simulink model "gm_untitled"  (R2020b)
settings: Solver=VariableStepAuto  StartTime=0.0  StopTime=0.001  RelTol=1e-3
libraries: simulink x1
settings Model: Creator=pablo  LastModifiedBy=pablo
settings OptimizationCC: BlockReduction=off  ConditionallyExecuteInputs=off
settings DebuggingCC: InheritedTsInSrcMsg=none

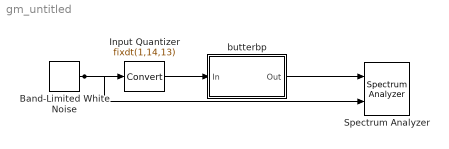
== system gm_untitled ==
  Band-Limited White Noise : simulink/Sources/Band-Limited White Noise  Cov=[0.1]  Ts=0.1  seed=[23341]
  Input Quantizer : DataTypeConversion  OutDataTypeStr=fixdt(1,14,13)  RndMeth=Round  SaturateOnIntegerOverflow=on
  Spectrum Analyzer : SpectrumAnalyzer  NumInputPorts=2
  butterbp : Subsystem
  wires:
  Band-Limited White Noise/1 -> Input Quantizer/1, Spectrum Analyzer/2
  butterbp/1(Out) -> Spectrum Analyzer/1
  Input Quantizer/1 -> butterbp/1(In)

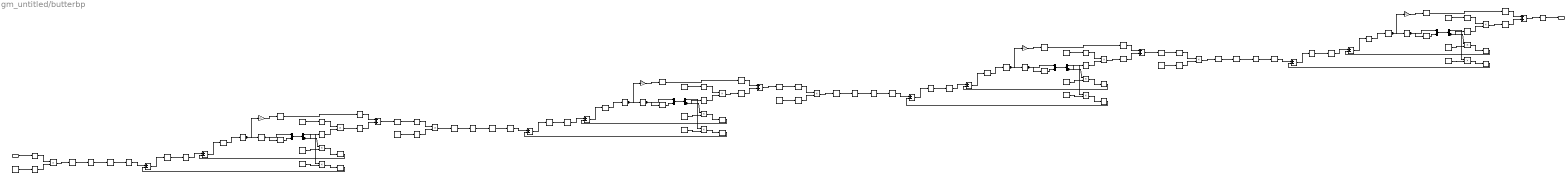
== system gm_untitled/butterbp ==
  In : Inport  OutDataTypeStr=fixdt(1, 14, 13)  PortDimensions=1  SampleTime=0.1
  HwModeRegister{,1..15} (16 alike) : Delay  DelayLength=double(1)  InitialCondition=0  SampleTime=0.1
  PipelineRegister{,1..7} (8 alike) : Delay  DelayLength=double(1)  InitialCondition=0  SampleTime=0.1
  Sub{,1..7} (8 alike) : Sum  Inputs=+-  OutDataTypeStr=fixdt(1, 41, 29)  RndMeth=Convergent  SampleTime=0.1
  adder{,1..3} (4 alike) : Sum  OutDataTypeStr=fixdt(1, 40, 29)  RndMeth=Convergent  SampleTime=0.1
  const : Constant  Value=0.009670734405517578125  OutDataTypeStr=fixdt(1, 16, 21)  SampleTime=0.1
  const1 : Constant  Value=-1.60137939453125  OutDataTypeStr=fixdt(1, 16, 14)  SampleTime=0.1
  const10 : Constant  Value=-1.60809326171875  OutDataTypeStr=fixdt(1, 16, 14)  SampleTime=0.1
  const11 : Constant  Value=0.9822998046875  OutDataTypeStr=fixdt(1, 16, 14)  SampleTime=0.1
  const2 : Constant  Value=0.99249267578125  OutDataTypeStr=fixdt(1, 16, 14)  SampleTime=0.1
  const3 : Constant  Value=0.009670734405517578125  OutDataTypeStr=fixdt(1, 16, 21)  SampleTime=0.1
  const4 : Constant  Value=-1.62249755859375  OutDataTypeStr=fixdt(1, 16, 14)  SampleTime=0.1
  const5 : Constant  Value=0.99267578125  OutDataTypeStr=fixdt(1, 16, 14)  SampleTime=0.1
  const6 : Constant  Value=0.00962066650390625  OutDataTypeStr=fixdt(1, 16, 21)  SampleTime=0.1
  const7 : Constant  Value=-1.5992431640625  OutDataTypeStr=fixdt(1, 16, 14)  SampleTime=0.1
  const8 : Constant  Value=0.98211669921875  OutDataTypeStr=fixdt(1, 16, 14)  SampleTime=0.1
  const9 : Constant  Value=0.00962066650390625  OutDataTypeStr=fixdt(1, 16, 21)  SampleTime=0.1
  delayMatch{,1..3} (4 alike) : Delay  DelayLength=double(2)  InitialCondition=0  SampleTime=0.1
  delay_process_section1_tap0 : Delay  DelayLength=double(1)  SampleTime=0.1
  delay_process_section1_tap1 : Delay  DelayLength=double(1)  SampleTime=0.1
  delay_process_section2_tap0 : Delay  DelayLength=double(1)  SampleTime=0.1
  delay_process_section2_tap1 : Delay  DelayLength=double(1)  SampleTime=0.1
  delay_process_section3_tap0 : Delay  DelayLength=double(1)  SampleTime=0.1
  delay_process_section3_tap1 : Delay  DelayLength=double(1)  SampleTime=0.1
  delay_process_section4_tap0 : Delay  DelayLength=double(1)  SampleTime=0.1
  delay_process_section4_tap1 : Delay  DelayLength=double(1)  SampleTime=0.1
  dtc{,4,8,12} (4 alike) : DataTypeConversion  OutDataTypeStr=fixdt(1, 16, 16)  RndMeth=Convergent  SampleTime=0.1
  dtc{1..2,5..6,9..10,13..14,16..20,22..26,28..32,34..38} (28 alike) : DataTypeConversion  OutDataTypeStr=fixdt(1, 40, 29)  RndMeth=Convergent  SampleTime=0.1
  dtc11 : DataTypeConversion  OutDataTypeStr=fixdt(1, 16, 11)  RndMeth=Convergent  SampleTime=0.1
  dtc15 : DataTypeConversion  OutDataTypeStr=fixdt(1, 18, 13)  RndMeth=Convergent  SampleTime=0.1
  dtc{21,27,33,39} (4 alike) : DataTypeConversion  OutDataTypeStr=fixdt(1, 16, 15)  RndMeth=Convergent  SampleTime=0.1
  dtc3 : DataTypeConversion  OutDataTypeStr=fixdt(1, 16, 11)  RndMeth=Convergent  SampleTime=0.1
  dtc7 : DataTypeConversion  OutDataTypeStr=fixdt(1, 16, 11)  RndMeth=Convergent  SampleTime=0.1
  gain{,1..3} (4 alike) : Gain  Gain="fi(0,1,16,14,\"hex\",\"4000\")"  ParamDataTypeStr=fixdt(1, 16, 14)  OutDataTypeStr=fixdt(1, 32, 29)  RndMeth=Convergent  SampleTime=0.1
  gain{4..7} (4 alike) : Product  Inputs=**  OutDataTypeStr=fixdt(1, 32, 29)  RndMeth=Convergent  SampleTime=0.1
  gain_const{,1..3} (4 alike) : Constant  Value=-1  OutDataTypeStr=fixdt(1, 16, 14)  SampleTime=0.1
  multiplier : Product  Inputs=**  OutDataTypeStr=fixdt(1, 30, 34)  SampleTime=0.1
  multiplier1 : Product  Inputs=**  OutDataTypeStr=fixdt(1, 32, 32)  SampleTime=0.1
  multiplier{4..11} (8 alike) : Product  Inputs=**  OutDataTypeStr=fixdt(1, 32, 29)  RndMeth=Convergent  SampleTime=0.1
  multiplier2 : Product  Inputs=**  OutDataTypeStr=fixdt(1, 32, 32)  SampleTime=0.1
  multiplier3 : Product  Inputs=**  OutDataTypeStr=fixdt(1, 32, 32)  SampleTime=0.1
  multiplier_out_dtc{,1..3} (4 alike) : DataTypeConversion  OutDataTypeStr=fixdt(1, 34, 34)  RndMeth=Convergent  SampleTime=0.1
  t{,2,4,6} (4 alike) : Mux  Inputs=2
  t{1,3,5,7} (4 alike) : Demux  Outputs=2
  Out : Outport
  wires:
  In/1 -> HwModeRegister/1
  const/1 -> HwModeRegister1/1
  multiplier_out_dtc/1 -> dtc/1
  const1/1 -> multiplier5/2
  const2/1 -> multiplier4/2
  dtc/1 -> dtc1/1
  adder/1 -> dtc3/1
  dtc1/1 -> Sub/1
  gain/1 -> dtc2/1
  PipelineRegister4/1 -> adder/2
  delayMatch/1 -> adder/1
  dtc3/1 -> HwModeRegister2/1
  const3/1 -> HwModeRegister3/1
  multiplier_out_dtc1/1 -> dtc4/1
  const4/1 -> multiplier7/2
  const5/1 -> multiplier6/2
  dtc4/1 -> dtc5/1
  adder1/1 -> dtc7/1
  dtc5/1 -> Sub2/1
  gain1/1 -> dtc6/1
  PipelineRegister5/1 -> adder1/2
  delayMatch1/1 -> adder1/1
  dtc7/1 -> HwModeRegister4/1
  const6/1 -> HwModeRegister5/1
  multiplier_out_dtc2/1 -> dtc8/1
  const7/1 -> multiplier9/2
  const8/1 -> multiplier8/2
  dtc8/1 -> dtc9/1
  adder2/1 -> dtc11/1
  dtc9/1 -> Sub4/1
  gain2/1 -> dtc10/1
  PipelineRegister6/1 -> adder2/2
  delayMatch2/1 -> adder2/1
  dtc11/1 -> HwModeRegister6/1
  const9/1 -> HwModeRegister7/1
  multiplier_out_dtc3/1 -> dtc12/1
  const10/1 -> multiplier11/2
  const11/1 -> multiplier10/2
  dtc12/1 -> dtc13/1
  adder3/1 -> dtc15/1
  dtc13/1 -> Sub6/1
  gain3/1 -> dtc14/1
  PipelineRegister7/1 -> adder3/2
  delayMatch3/1 -> adder3/1
  dtc15/1 -> Out/1
  gain_const/1 -> HwModeRegister8/1
  gain_const1/1 -> HwModeRegister10/1
  gain_const2/1 -> HwModeRegister12/1
  gain_const3/1 -> HwModeRegister14/1
  PipelineRegister/1 -> multiplier_out_dtc/1
  PipelineRegister1/1 -> multiplier_out_dtc1/1
  PipelineRegister2/1 -> multiplier_out_dtc2/1
  PipelineRegister3/1 -> multiplier_out_dtc3/1
  dtc2/1 -> delayMatch/1
  dtc6/1 -> delayMatch1/1
  dtc10/1 -> delayMatch2/1
  dtc14/1 -> delayMatch3/1
  multiplier4/1 -> dtc16/1
  dtc16/1 -> Sub1/2
  delay_process_section1_tap1/1 -> t/2
  delay_process_section1_tap0/1 -> delay_process_section1_tap1/1, t/1
  t/1 -> t1/1
  t1/1 -> multiplier5/1
  multiplier5/1 -> dtc17/1
  dtc17/1 -> Sub/2
  Sub/1 -> dtc18/1
  dtc18/1 -> dtc19/1
  dtc19/1 -> Sub1/1
  Sub1/1 -> dtc20/1
  dtc20/1 -> dtc21/1
  t1/2 -> multiplier4/1, HwModeRegister9/1
  dtc21/1 -> delay_process_section1_tap0/1, gain/1
  multiplier6/1 -> dtc22/1
  dtc22/1 -> Sub3/2
  delay_process_section2_tap1/1 -> t2/2
  delay_process_section2_tap0/1 -> delay_process_section2_tap1/1, t2/1
  t2/1 -> t3/1
  t3/1 -> multiplier7/1
  multiplier7/1 -> dtc23/1
  dtc23/1 -> Sub2/2
  Sub2/1 -> dtc24/1
  dtc24/1 -> dtc25/1
  dtc25/1 -> Sub3/1
  Sub3/1 -> dtc26/1
  dtc26/1 -> dtc27/1
  t3/2 -> multiplier6/1, HwModeRegister11/1
  dtc27/1 -> delay_process_section2_tap0/1, gain1/1
  multiplier8/1 -> dtc28/1
  dtc28/1 -> Sub5/2
  delay_process_section3_tap1/1 -> t4/2
  delay_process_section3_tap0/1 -> delay_process_section3_tap1/1, t4/1
  t4/1 -> t5/1
  t5/1 -> multiplier9/1
  multiplier9/1 -> dtc29/1
  dtc29/1 -> Sub4/2
  Sub4/1 -> dtc30/1
  dtc30/1 -> dtc31/1
  dtc31/1 -> Sub5/1
  Sub5/1 -> dtc32/1
  dtc32/1 -> dtc33/1
  t5/2 -> multiplier8/1, HwModeRegister13/1
  dtc33/1 -> delay_process_section3_tap0/1, gain2/1
  multiplier10/1 -> dtc34/1
  dtc34/1 -> Sub7/2
  delay_process_section4_tap1/1 -> t6/2
  delay_process_section4_tap0/1 -> delay_process_section4_tap1/1, t6/1
  t6/1 -> t7/1
  t7/1 -> multiplier11/1
  multiplier11/1 -> dtc35/1
  dtc35/1 -> Sub6/2
  Sub6/1 -> dtc36/1
  dtc36/1 -> dtc37/1
  dtc37/1 -> Sub7/1
  Sub7/1 -> dtc38/1
  dtc38/1 -> dtc39/1
  t7/2 -> multiplier10/1, HwModeRegister15/1
  dtc39/1 -> delay_process_section4_tap0/1, gain3/1
  multiplier/1 -> PipelineRegister/1
  HwModeRegister/1 -> multiplier/1
  HwModeRegister1/1 -> multiplier/2
  multiplier1/1 -> PipelineRegister1/1
  HwModeRegister2/1 -> multiplier1/1
  HwModeRegister3/1 -> multiplier1/2
  multiplier2/1 -> PipelineRegister2/1
  HwModeRegister4/1 -> multiplier2/1
  HwModeRegister5/1 -> multiplier2/2
  multiplier3/1 -> PipelineRegister3/1
  HwModeRegister6/1 -> multiplier3/1
  HwModeRegister7/1 -> multiplier3/2
  gain4/1 -> PipelineRegister4/1
  HwModeRegister8/1 -> gain4/1
  HwModeRegister9/1 -> gain4/2
  gain5/1 -> PipelineRegister5/1
  HwModeRegister10/1 -> gain5/1
  HwModeRegister11/1 -> gain5/2
  gain6/1 -> PipelineRegister6/1
  HwModeRegister12/1 -> gain6/1
  HwModeRegister13/1 -> gain6/2
  gain7/1 -> PipelineRegister7/1
  HwModeRegister14/1 -> gain7/1
  HwModeRegister15/1 -> gain7/2
